simulink model "essai_5"  (R2016a)
settings: Solver=ode15s  StartTime=0.0  StopTime=1e9  RelTol=1e-3
libraries: nesl_utility x63, simCryogenics_lib x62, fl_lib x6
settings Model: Creator=FB229602  LastModifiedBy=FB229602
settings DataIOCC: LimitDataPoints=on  SaveFormat=Array
settings DebuggingCC: ParameterTunabilityLossMsg=none
settings HardwareCC: ProdBitPerInt=16  ProdBitPerPointer=16  ProdLargestAtomicFloat=None  ProdIntDivRoundTo=Undefined  ProdEndianess=Unspecified  ProdWordSize=16  ProdHWDeviceType=Generic->16-bit Embedded Processor  TargetBitPerPointer=64  TargetLongLongMode=on  TargetIntDivRoundTo=Zero  TargetEndianess=LittleEndian  TargetWordSize=64  TargetHWDeviceType=MATLAB Host  ProdEqTarget=off
settings ModelReferenceCC: PropagateSignalLabelsOutOfModel=off
settings ConfigComp: CovModelRefEnable=Off
settings SimscapeCC: SimscapeLogType=all

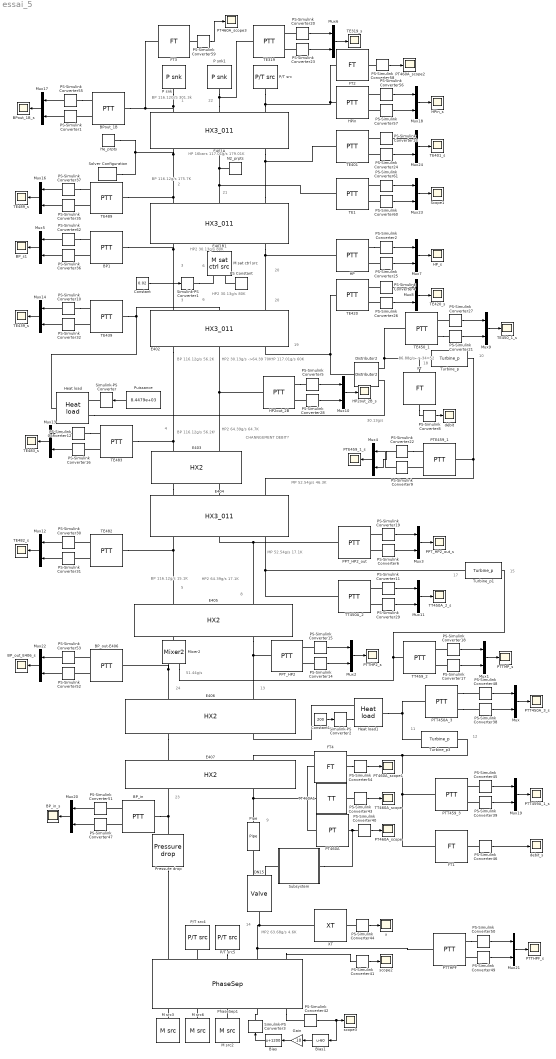
== system essai_5 ==
  note: 18
  note: 10
  note: 17
  note: 15
  note: 13
  note: 8
  note: 7
  note: 6
  note: 19
  note: 20
  note: 24
  note: 5
  note: 4
  note: 3
  note: MP
      | 52.54g/s
      | 17.1K
  note: HP2
      | 64.39g/s
      | 17.1K
  note: BP
      | 116.12g/s
      | 15.1K
  note: MP
      | 52.54g/s
      | 46.3K
  note: CHANNGEMENT DEBIT?
  note: HP2
      | 64.39g/s
      | 64.7K
  note: BP
      | 116.12g/s
      | 56.2K
  note: 30.13g/s
  note: 86.88g/s
      | ->-34=52
  note: HP
      | 117.01g/s
      | 60K
  note: HP2
      | 30.13g/s ->64.39
      | 70K
  note: BP
      | 116.12g/s
      | 56.2K
  note: HP2
      | 30.13g/s
      | 80K
  note: 51.44g/s
  note: 9
  note: 14
  note: 11
  note: 12
  note: 23
  note: MP2
      | 63.68g/s
      | 4.6K
  note: 6
  note: 20
  note: 21
  note: 22
  note: 3
  note: 2
  note: 1
  note: BP
      | 116.12G/S
      | 301.3k
  note: HP
      | 16bars
      | 117.01g/s
      | 179.01K
  note: BP
      | 116.12g/s
      | 175.7K
  note: HP2
      | 30.13g/s
      | 80K
  BP1 : simCryogenics_lib/Sensors/PTT
  BP_in : simCryogenics_lib/Sensors/PTT
  "BP_in_s " : Scope
  BP_out-E406 : simCryogenics_lib/Sensors/PTT
  BP_out_E406_s : Scope
  BP_s1 : Scope
  BPout_1B : simCryogenics_lib/Sensors/PTT
  BPout_1B_s : Scope
  Bias : Bias  Bias=1200
  Bias1 : Bias  Bias=-60
  Constant : Constant  Value=0.02
  Constant1 : Constant  Value=200
  "DN15 " : simCryogenics_lib/Elements/Valve  CVmax=1.5  ControlInputMin=0  ControlInputMax=100  Xt=0.86  Rv=10  lin_v=0  lim_v=0  K=2.4e-5 m^1.50000*kg^0.50000/s/bar^0.50000  Cmd_specify=off  Cmd_priority=High  Cmd=0  gamma_specify=off  gamma_priority=High  gamma=0  rho_specify=off  rho_priority=High  rho=0 kg/m^3  Xc_specify=off  Xc_priority=High  Xc=0  X_specify=off  X_priority=High  X=0  Y_specify=off  Y_priority=High  Y=0  CV_specify=off  CV_priority=High  CV=0
  Distributor2 : simCryogenics_lib/Elements/Distributor2
  E401A : simCryogenics_lib/Elements/HX3_011  N=9  Vh=0.118 m^3  Vm=0.055 m^3  Vc=0.008 km^3  M=281 kg  Kh=0.062/0.11612 s*bar/kg  Km=0.033/0.11701 s*bar/kg  Kc=0.021/0.11701 s*bar/kg  hh_m=0 J/s/K  hh_c=2.5e4 J/s/K  hm_c=250 J/s/K  Th0=300 K  Ph0=15 bar  Mh0=0.11612 kg/s  Tm0=175 K  Pm0=1 bar  Mm0=0.0026 kg/s  Tc0=175.7 K  Pc0=1.05 bar  Mc0=0.11612 kg/s  sensh=0  sensm=1  sensc=1
  E401B1 : simCryogenics_lib/Elements/HX3_011  N=9  Vh=0.133 m^3  Vm=0.062 m^3  Vc=0.012 m^3  M=195 kg  Kh=0.0255/0.11612 s*bar/kg  Km=0.014/0.11701 s*bar/kg  Kc=0.002/0.11701 s*bar/kg  hh_m=5000 J/s/K  hh_c=3e4 J/s/K  hm_c=1 J/s/K  Th0=179 K  Ph0=14.4 bar  Mh0=0.116 kg/s  Tm0=79 K  Pm0=1.1 bar  Mm0=0.0026 kg/s  Tc0=79.2 K  Pc0=1.05 bar  Mc0=0.116 kg/s  sensh=0  sensm=1  sensc=1
  E402 : simCryogenics_lib/Elements/HX3_011  N=9  Vh=0.133 m^3  Vm=0.005 m^3  Vc=0.012 m^3  M=195 kg  Kh=0.0255/0.11612 s*bar/kg  Km=0.011/0.03013 s*bar/kg  Kc=0.014/0.11701 s*bar/kg  hh_m=8000 J/s/K  hh_c=8000 J/s/K  hm_c=1 J/s/K  Th0=56.2 K  Ph0=1.05 bar  Mh0=0.11612 kg/s  Tm0=80 K  Pm0=14.73 bar  Mm0=0.06439 kg/s  Tc0=100 K  Pc0=14.73 bar  Mc0=0.11701 kg/s  sensh=0  sensm=1  sensc=1
  E403 : simCryogenics_lib/Elements/HX2  N=9  Vh=0.049 m^3  Vc=0.172 m^3  M=227.5 kg  Kh=0.003/0.06439 s*bar/kg  Kc=0.0055/0.11612 s*bar/kg  h=5700 J/s/K  Th0=64.7 K  Ph0=14.73 bar  Mh0=0.116 kg/s  Tc0=46 K  Pc0=1.05 bar  Mc0=0.064 kg/s
  E404 : simCryogenics_lib/Elements/HX3_011  N=9  Vh=0.172 m^3  Vm=0.049 m^3  Vc=0.045 m^3  M=227.5 kg  Kh=0.0055/0.011612 s*bar/kg  Km=0.003/0.06439 s*bar/kg  Kc=0.004/0.05254 s*bar/kg  hh_m=11000 J/s/K  hh_c=8000 J/s/K  hm_c=1 J/s/K  Th0=15.1 K  Ph0=1.05 bar  Mh0=0.116 kg/s  Tm0=46 K  Pm0=14.73 bar  Mm0=0.064 kg/s  Tc0=46.3 K  Pc0=5 bar  Mc0=0.052 kg/s  sensh=0  sensm=1  sensc=1
  "E405 " : simCryogenics_lib/Elements/HX2  N=9  Vh=0.023 m^3  Vc=0.065 m^3  M=64 kg  Kh=0.001/0.6439 s*bar/kg  Kc=0.0023/0.11612 s*bar/kg  h=1500 J/s/K  Th0=17.1 K  Ph0=14.73 bar  Mh0=0.11612 kg/s  Tc0=10 K  Pc0=1.05 bar  Mc0=0.06439 kg/s
  E406 : simCryogenics_lib/Elements/HX2  N=9  Vh=0.065 m^3  Vc=0.023 m^3  M=64 kg  Kh=0.001/0.06439 s*bar/kg  Kc=0.0023/0.06368 s*bar/kg  h=1000 J/s/K  Th0=17 K  Ph0=14.73 bar  Mh0=0.06368 kg/s  Tc0=5 K  Pc0=1.05 bar  Mc0=0.06439 kg/s
  E407 : simCryogenics_lib/Elements/HX2  N=9  Vh=0.011 m^3  Vc=0.065 m^3  M=64 kg  Kh=0.002/0.06368 s*bar/kg  Kc=0.0023/0.06368 s*bar/kg  h=2000 J/s/K  Th0=5.7 K  Ph0=3.03 bar  Mh0=0.06368 kg/s  Tc0=4.4 K  Pc0=1.05 bar  Mc0=0.06368 kg/s
  FT{,1..4} (5 alike) : simCryogenics_lib/Sensors/FT
  Gain : Gain  Gain=10
  HP : simCryogenics_lib/Sensors/PTT
  HP2out_2B : simCryogenics_lib/Sensors/PTT
  HP2out_2B_s : Scope
  HP_s : Scope
  HPin : simCryogenics_lib/Sensors/PTT
  HPin_s : Scope
  He_prpts : simCryogenics_lib/Utilities/He_prpts  P_min=0.1 bar  P_max=30 bar  T_min=3 K  T_max=320 K  N=100  Mol=4.0026 * 10 ^ (- 3) kg/mol
  Heat load : simCryogenics_lib/Utilities/Heat load
  Heat load1 : simCryogenics_lib/Utilities/Heat load
  M sat ctrl src : simCryogenics_lib/Sources_Sinks/M sat ctrl src
  M src2 : simCryogenics_lib/Sources_Sinks/M src  M=0 kg/s
  M src3 : simCryogenics_lib/Sources_Sinks/M src  M=0 kg/s
  M src6 : simCryogenics_lib/Sources_Sinks/M src  M=0 kg/s
  Mixer2 : simCryogenics_lib/Elements/Mixer2
  Mux{,1..14,16..24} (24 alike) : Mux  Inputs=2
  N2_prpts : simCryogenics_lib/Utilities/N2_prpts  P_min=0.5 bar  T_min=70 K  T_max=320 K  P_max=20 bar  Mol=4.0026 * (10 ^ (- 3)) kg/mol
  P snk : simCryogenics_lib/Sources_Sinks/P snk  P=1.05 bar
  P snk1 : simCryogenics_lib/Sources_Sinks/P snk  P=1.05 bar
  P/T src : simCryogenics_lib/Sources_Sinks/P//T src  P=14.73 bar  T=305 K
  P/T src4 : simCryogenics_lib/Sources_Sinks/P//T src  P=5 bar  T=46.3 K
  P/T src5 : simCryogenics_lib/Sources_Sinks/P//T src  P=5 bar  T=46.3 K
  PPT_HP2 : simCryogenics_lib/Sensors/PTT
  PPT_HP2_out : simCryogenics_lib/Sensors/PTT
  PPT_HP2_out_s : Scope
  PS Constant : fl_lib/Physical Signals/Sources/PS Constant  constant=0
  PS-Simulink Converter{1..2,4..6,8..32,35..62} (58 alike) : nesl_utility/PS-Simulink Converter  PhysicalDomain=network_engine_domain  SubClassName=ps_output  LeftPortType=input  RightPortType=output  PseudoPeriodic=off  Frequencies=[]  Unit=1  AffineConversion=off
  PT460A : simCryogenics_lib/Sensors/PT
  PT460A_scope{,1..3} (4 alike) : Scope
  PTE459_1 : simCryogenics_lib/Sensors/PTT
  PTE459_1_s : Scope
  PTT450A_3 : simCryogenics_lib/Sensors/PTT
  PTT450A_3_s : Scope
  PTT459A_1_s : Scope
  PTT459_3 : simCryogenics_lib/Sensors/PTT
  PTTHP2_s : Scope
  PTTHPF : simCryogenics_lib/Sensors/PTT
  PTTHPF_s : Scope
  PTTMP_s : Scope
  PhaseSep1 : simCryogenics_lib/Elements/PhaseSep  Ideal1=1  DeltaT1=0.05 K  N1=10  h1=400 W/K  Ideal2=1  DeltaT2=0.05 K  N2=10  h2=400 W/K  hmax=1.601 m  S=3.4636 m^2  P0=1.3 bar  h0=20  T0=4.5 K
  Pipe : simCryogenics_lib/Elements/Pipe  Vol=0.01 m^3  Ideal=0  P0=3 bar  T0=4.6 K
  Pressure drop : simCryogenics_lib/Utilities/Pressure drop  K=0.10/0.065 s*bar/kg
  "Puissance " : Constant  Value=8.4479e+03
  Scope1 : Scope
  Simulink-PS Converter{,1..3} (4 alike) : nesl_utility/Simulink-PS Converter  PhysicalDomain=network_engine_domain  SubClassName=ps_input  LeftPortType=input  RightPortType=output  PseudoPeriodic=off  Frequencies=[]  NoiseDistribution=none  NoiseParameters=[]  Unit=1  AffineConversion=off  InputFiltering=off  SimscapeFilterOrder=1  InputFilterTimeConstant=0.001  UdotUserProvided=1
  Solver Configuration : nesl_utility/Solver Configuration  PhysicalDomain=network_engine_domain  SubClassName=solver  LeftPortType=input  RightPortType=generic  Accelerate=off  Tones=[]  Harmonics=[]  SimulateNoise=off  Profile=off  UseLocalSampling=off  EnableSwitchedLinearOptims=on  FrequencyDomain=off  UseCCode=off  RelTol=0.001  AbsTol=1e-06  MinStep=1e-09  ToWorkspace=off  RevertToSquareIcSolve=off  NumHomotopyIterations=100  PhasorMode=off  PhasorModeNumHarmonics=1  OverrideAbsTol=off  DoDC=off  ResidualTolerance=1e-09  UseLocalSolver=off  LocalSolverChoice=NE_BACKWARD_EULER_ADVANCER  LocalSolverSampleTime=0.001  DoFixedCost=off  MaxNonlinIter=3  MaxModeIter=2  LinearAlgebra=Sparse  DelaysMemoryBudget=1024  AutomaticFiltering=on  FilteringTimeConstant=0.001
  Subsystem : Subsystem
  TE{1,319,401,420,439,482..483,489} (8 alike) : simCryogenics_lib/Sensors/PTT
  TE319_s : Scope
  TE401_s : Scope
  TE420_s : Scope
  TE439_s : Scope
  TE450_1 : simCryogenics_lib/Sensors/PTT
  TE450_1_s : Scope
  TE482_s : Scope
  TE483_s : Scope
  TE489_s : Scope
  TT450A_2 : simCryogenics_lib/Sensors/PTT
  TT450A_2_s : Scope
  TT459_2 : simCryogenics_lib/Sensors/PTT
  TT460A1 : simCryogenics_lib/Sensors/TT
  TT460A_scope : Scope
  Turbine_p : simCryogenics_lib/Elements/Turbine_p  A=2.5747e-05 m^2  D=0.05 m  Mass=0.02 kg  cst_eff=1  eta0=0.75  Tin0=60 K  Pin0=14.73 bar  Pout0=5 bar  N0=2250 1/s  Q0=0 W  v0=0  I=0 kg*m^2  gamma_specify=off  gamma_priority=High  gamma=0  C_specify=off  C_priority=High  C=0  Z_specify=off  Z_priority=High  Z=0  Cp_specify=off  Cp_priority=High  Cp=0 kJ/kg/K  Sin_specify=off  Sin_priority=High  Sin=0 kJ/kg  T_specify=off  T_priority=High  T=0 K  HoutIs_specify=off  HoutIs_priority=High  HoutIs=0 kJ/kg  u1_specify=off  u1_priority=High  u1=0 m/s  c1_specify=off  c1_priority=High  c1=0 m/s  v_specify=off  v_priority=High  v=0  eta_specify=off  eta_priority=High  eta=0  eta_var_specify=off  eta_var_priority=High  eta_var=0  N_specify=off  N_priority=High  N=0 rad/s  Q_specify=off  Q_priority=High  Q=0 W
  Turbine_p1 : simCryogenics_lib/Elements/Turbine_p  A=2.6523e-05 m^2  D=0.02 m  Mass=0.02 kg  cst_eff=1  eta0=0.75  Tin0=17.1 K  Pin0=5 bar  Pout0=1.3 bar  N0=2250 1/s  Q0=0 W  v0=0  I=0 kg*m^2  gamma_specify=off  gamma_priority=High  gamma=0  C_specify=off  C_priority=High  C=0  Z_specify=off  Z_priority=High  Z=0  Cp_specify=off  Cp_priority=High  Cp=0 kJ/kg/K  Sin_specify=off  Sin_priority=High  Sin=0 kJ/kg  T_specify=off  T_priority=High  T=0 K  HoutIs_specify=off  HoutIs_priority=High  HoutIs=0 kJ/kg  u1_specify=off  u1_priority=High  u1=0 m/s  c1_specify=off  c1_priority=High  c1=0 m/s  v_specify=off  v_priority=High  v=0  eta_specify=off  eta_priority=High  eta=0  eta_var_specify=off  eta_var_priority=High  eta_var=0  N_specify=off  N_priority=High  N=0 rad/s  Q_specify=off  Q_priority=High  Q=0 W
  Turbine_p3 : simCryogenics_lib/Elements/Turbine_p  A=6.0851e-06 m^2  D=0.01 m  Mass=0.02 kg  cst_eff=0  eta0=0.75  Tin0=7.19 K  Pin0=14.73 bar  Pout0=3.03 bar  N0=2250 1/s  Q0=0 W  v0=0  I=0 kg*m^2  gamma_specify=off  gamma_priority=High  gamma=0  C_specify=off  C_priority=High  C=0  Z_specify=off  Z_priority=High  Z=0  Cp_specify=off  Cp_priority=High  Cp=0 kJ/kg/K  Sin_specify=off  Sin_priority=High  Sin=0 kJ/kg  T_specify=off  T_priority=High  T=0 K  HoutIs_specify=off  HoutIs_priority=High  HoutIs=0 kJ/kg  u1_specify=off  u1_priority=High  u1=0 m/s  c1_specify=off  c1_priority=High  c1=0 m/s  v_specify=off  v_priority=High  v=0  eta_specify=off  eta_priority=High  eta=0  eta_var_specify=off  eta_var_priority=High  eta_var=0  N_specify=off  N_priority=High  N=0 rad/s  Q_specify=off  Q_priority=High  Q=0 W
  XT : simCryogenics_lib/Sensors/XT
  debit_s : Scope
  débit : Scope
  scope2 : Scope
  scope3 : Scope
  x : Scope
  wires:
  "Puissance "/1 -> Simulink-PS Converter/1
  PS-Simulink Converter8/1 -> débit/1
  PS-Simulink Converter15/1 -> Mux2/1
  PS-Simulink Converter14/1 -> Mux2/2
  Mux2/1 -> PTTHP2_s/1
  PS-Simulink Converter18/1 -> Mux1/1
  PS-Simulink Converter17/1 -> Mux1/2
  Mux1/1 -> PTTMP_s/1
  PS-Simulink Converter19/1 -> Mux3/1
  PS-Simulink Converter6/1 -> Mux3/2
  Mux3/1 -> PPT_HP2_out_s/1
  Mux4/1 -> PTE459_1_s/1
  PS-Simulink Converter25/1 -> Mux7/2
  Mux7/1 -> HP_s/1
  PS-Simulink Converter4/1 -> Mux8/1
  PS-Simulink Converter26/1 -> Mux8/2
  Mux8/1 -> TE420_s/1
  PS-Simulink Converter27/1 -> Mux9/1
  Mux9/1 -> TE450_1_s/1
  PS-Simulink Converter2/1 -> Mux7/1
  PS-Simulink Converter28/1 -> Mux10/2
  Mux10/1 -> HP2out_2B_s/1
  PS-Simulink Converter5/1 -> Mux10/1
  PS-Simulink Converter11/1 -> Mux11/1
  PS-Simulink Converter29/1 -> Mux11/2
  Mux11/1 -> TT450A_2_s/1
  Mux12/1 -> TE482_s/1
  PS-Simulink Converter30/1 -> Mux12/1
  PS-Simulink Converter31/1 -> Mux12/2
  Mux13/1 -> TE483_s/1
  PS-Simulink Converter12/1 -> Mux13/1
  PS-Simulink Converter16/1 -> Mux13/2
  Mux14/1 -> TE439_s/1
  PS-Simulink Converter10/1 -> Mux14/1
  PS-Simulink Converter32/1 -> Mux14/2
  PS-Simulink Converter9/1 -> Mux4/1
  PS-Simulink Converter22/1 -> Mux4/2
  PS-Simulink Converter21/1 -> Mux9/2
  Bias/1 -> Simulink-PS Converter3/1
  PS-Simulink Converter46/1 -> debit_s/1
  PS-Simulink Converter40/1 -> PT460A_scope/1
  PS-Simulink Converter43/1 -> TT460A_scope/1
  PS-Simulink Converter44/1 -> x/1
  PS-Simulink Converter48/1 -> Mux/1
  PS-Simulink Converter42/1 -> Bias1/1, scope3/1
  Gain/1 -> Bias/1
  Bias1/1 -> Gain/1
  PS-Simulink Converter38/1 -> Mux/2
  Mux/1 -> PTT450A_3_s/1
  PS-Simulink Converter45/1 -> Mux19/1
  PS-Simulink Converter39/1 -> Mux19/2
  Mux19/1 -> PTT459A_1_s/1
  PS-Simulink Converter50/1 -> Mux21/1
  PS-Simulink Converter49/1 -> Mux21/2
  Mux21/1 -> PTTHPF_s/1
  Mux20/1 -> "BP_in_s "/1
  PS-Simulink Converter51/1 -> Mux20/1
  PS-Simulink Converter47/1 -> Mux20/2
  Mux22/1 -> BP_out_E406_s/1
  PS-Simulink Converter53/1 -> Mux22/1
  PS-Simulink Converter52/1 -> Mux22/2
  PS-Simulink Converter41/1 -> scope2/1
  PS-Simulink Converter54/1 -> PT460A_scope1/1
  PS-Simulink Converter20/1 -> Mux6/1
  PS-Simulink Converter23/1 -> Mux6/2
  Mux6/1 -> TE319_s/1
  PS-Simulink Converter13/1 -> Mux24/1
  PS-Simulink Converter24/1 -> Mux24/2
  Mux24/1 -> TE401_s/1
  Mux5/1 -> BP_s1/1
  PS-Simulink Converter62/1 -> Mux5/1
  PS-Simulink Converter36/1 -> Mux5/2
  Mux16/1 -> TE489_s/1
  PS-Simulink Converter37/1 -> Mux16/1
  PS-Simulink Converter35/1 -> Mux16/2
  Mux17/1 -> BPout_1B_s/1
  PS-Simulink Converter55/1 -> Mux17/1
  PS-Simulink Converter1/1 -> Mux17/2
  PS-Simulink Converter56/1 -> Mux18/1
  PS-Simulink Converter57/1 -> Mux18/2
  Mux18/1 -> HPin_s/1
  PS-Simulink Converter58/1 -> PT460A_scope2/1
  PS-Simulink Converter59/1 -> PT460A_scope3/1
  PS-Simulink Converter60/1 -> Mux23/2
  Mux23/1 -> Scope1/1
  PS-Simulink Converter61/1 -> Mux23/1
  Constant/1 -> Simulink-PS Converter1/1
  Constant1/1 -> Simulink-PS Converter2/1
  connections:
  "E405 "/LConn1 -- E404/LConn3 -- TE482/LConn1
  E402/LConn3 -- E403/LConn1 -- TE483/LConn1
  E402/LConn2 -- E403/LConn2 -- HP2out_2B/LConn1
  "E405 "/LConn2 -- E404/LConn2 -- PPT_HP2_out/LConn1
  TT450A_2/LConn1 -- E404/LConn1 -- Turbine_p1/LConn1
  Turbine_p/RConn1 -- E404/RConn1 -- PTE459_1/LConn1
  E401B1/RConn1 -- E402/RConn3 -- BP1/LConn1
  HP/LConn1 -- E401B1/RConn3 -- E402/RConn1
  Distributor2/LConn1 -- TE420/LConn1 -- E402/LConn1
  Heat load/RConn1 -- TE439/LConn1 -- E402/RConn2
  FT/LConn1 -- TE450_1/LConn1 -- Distributor2/RConn1 -- Turbine_p/LConn1
  Heat load/LConn1 -- Distributor2/RConn2
  Simulink-PS Converter/RConn1 -- Heat load/LConn2
  FT/RConn1 -- PS-Simulink Converter8/LConn1
  Mixer2/RConn1 -- "E405 "/RConn1
  Mixer2/LConn2 -- TT459_2/LConn1 -- Turbine_p1/RConn1
  PS-Simulink Converter14/LConn1 -- PPT_HP2/RConn2
  PS-Simulink Converter15/LConn1 -- PPT_HP2/RConn1
  PS-Simulink Converter17/LConn1 -- TT459_2/RConn2
  PS-Simulink Converter18/LConn1 -- TT459_2/RConn1
  PS-Simulink Converter19/LConn1 -- PPT_HP2_out/RConn1
  PS-Simulink Converter6/LConn1 -- PPT_HP2_out/RConn2
  PS-Simulink Converter22/LConn1 -- PTE459_1/RConn2
  PTE459_1/RConn1 -- PS-Simulink Converter9/LConn1
  PS-Simulink Converter25/LConn1 -- HP/RConn2
  PS-Simulink Converter4/LConn1 -- TE420/RConn1
  PS-Simulink Converter26/LConn1 -- TE420/RConn2
  PS-Simulink Converter27/LConn1 -- TE450_1/RConn1
  HP/RConn1 -- PS-Simulink Converter2/LConn1
  HP2out_2B/RConn1 -- PS-Simulink Converter5/LConn1
  PS-Simulink Converter28/LConn1 -- HP2out_2B/RConn2
  PS-Simulink Converter29/LConn1 -- TT450A_2/RConn2
  PS-Simulink Converter11/LConn1 -- TT450A_2/RConn1
  TE450_1/RConn2 -- PS-Simulink Converter21/LConn1
  TE482/RConn1 -- PS-Simulink Converter30/LConn1
  TE482/RConn2 -- PS-Simulink Converter31/LConn1
  TE483/RConn2 -- PS-Simulink Converter16/LConn1
  PS-Simulink Converter12/LConn1 -- TE483/RConn1
  TE439/RConn2 -- PS-Simulink Converter32/LConn1
  PS-Simulink Converter10/LConn1 -- TE439/RConn1
  E407/RConn1 -- Pressure drop/RConn1 -- BP_in/LConn1
  PT460A/LConn1 -- FT4/LConn1 -- E407/RConn2 -- Pipe/LConn1 -- TT460A1/LConn1
  PTT450A_3/LConn1 -- Turbine_p3/LConn1 -- Heat load1/RConn1
  PTT459_3/LConn1 -- FT1/LConn1 -- Turbine_p3/RConn1 -- E407/LConn2
  "DN15 "/RConn1 -- PhaseSep1/LConn4 -- PTTHPF/LConn1 -- XT/LConn1
  PhaseSep1/LConn5 -- PS-Simulink Converter41/LConn1
  BP_in/RConn1 -- PS-Simulink Converter51/LConn1
  BP_out-E406/RConn1 -- PS-Simulink Converter53/LConn1
  PS-Simulink Converter44/LConn1 -- XT/RConn1
  PT460A/RConn1 -- Subsystem/RConn1 -- PS-Simulink Converter40/LConn1
  E406/RConn1 -- E407/LConn1
  PhaseSep1/LConn2 -- P/T src4/RConn1
  M src2/RConn1 -- PhaseSep1/RConn3
  BP_in/RConn2 -- PS-Simulink Converter47/LConn1
  "E405 "/RConn2 -- E406/LConn2 -- PPT_HP2/LConn1
  P/T src5/RConn1 -- PhaseSep1/LConn3
  PS-Simulink Converter39/LConn1 -- PTT459_3/RConn2
  PS-Simulink Converter46/LConn1 -- FT1/RConn1
  PS-Simulink Converter49/LConn1 -- PTTHPF/RConn2
  PTT450A_3/RConn1 -- PS-Simulink Converter48/LConn1
  PS-Simulink Converter43/LConn1 -- TT460A1/RConn1
  "DN15 "/LConn2 -- Pipe/RConn1
  M src6/RConn1 -- PhaseSep1/RConn2
  Simulink-PS Converter3/RConn1 -- PhaseSep1/RConn4
  PhaseSep1/RConn5 -- PS-Simulink Converter42/LConn1
  M src3/RConn1 -- PhaseSep1/RConn1
  PS-Simulink Converter45/LConn1 -- PTT459_3/RConn1
  PTT450A_3/RConn2 -- PS-Simulink Converter38/LConn1
  E406/LConn1 -- BP_out-E406/LConn1 -- Mixer2/LConn1
  E403/RConn1 -- E404/RConn3
  E403/RConn2 -- E404/RConn2
  BP_out-E406/RConn2 -- PS-Simulink Converter52/LConn1
  PTTHPF/RConn1 -- PS-Simulink Converter50/LConn1
  Pressure drop/LConn1 -- PhaseSep1/LConn1
  FT4/RConn1 -- PS-Simulink Converter54/LConn1
  Subsystem/LConn1 -- "DN15 "/LConn1
  FT3/LConn1 -- BPout_1B/LConn1 -- P snk/RConn1 -- E401A/LConn1
  E401A/RConn1 -- He_prpts/RConn1 -- Solver Configuration/RConn1 -- E401B1/LConn1 -- TE489/LConn1
  E401A/LConn3 -- FT2/LConn1 -- HPin/LConn1 -- P/T src/RConn1
  E401B1/LConn3 -- E401A/RConn3 -- TE401/LConn1
  E401A/LConn2 -- TE319/LConn1 -- P snk1/RConn1
  N2_prpts/RConn1 -- E401A/RConn2 -- E401B1/LConn2 -- TE1/LConn1
  PS-Simulink Converter56/LConn1 -- HPin/RConn1
  PS-Simulink Converter13/LConn1 -- TE401/RConn1
  BPout_1B/RConn2 -- PS-Simulink Converter1/LConn1
  PS-Simulink Converter37/LConn1 -- TE489/RConn1
  PS-Simulink Converter23/LConn1 -- TE319/RConn2
  PS-Simulink Converter60/LConn1 -- TE1/RConn2
  PS-Simulink Converter61/LConn1 -- TE1/RConn1
  PS-Simulink Converter20/LConn1 -- TE319/RConn1
  PS-Simulink Converter59/LConn1 -- FT3/RConn1
  PS-Simulink Converter24/LConn1 -- TE401/RConn2
  PS-Simulink Converter55/LConn1 -- BPout_1B/RConn1
  TE489/RConn2 -- PS-Simulink Converter35/LConn1
  M sat ctrl src/RConn1 -- E401B1/RConn2
  PS-Simulink Converter57/LConn1 -- HPin/RConn2
  PS-Simulink Converter58/LConn1 -- FT2/RConn1
  PS-Simulink Converter62/LConn1 -- BP1/RConn1
  BP1/RConn2 -- PS-Simulink Converter36/LConn1
  Simulink-PS Converter1/RConn1 -- M sat ctrl src/LConn1
  PS Constant/RConn1 -- M sat ctrl src/LConn2
  Heat load1/LConn1 -- E406/RConn2
  Simulink-PS Converter2/RConn1 -- Heat load1/LConn2

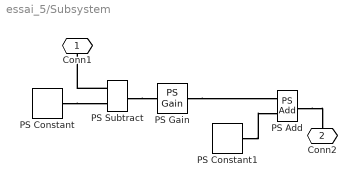
== system essai_5/Subsystem ==
  PS Add : fl_lib/Physical Signals/Functions/PS Add
  PS Constant : fl_lib/Physical Signals/Sources/PS Constant  constant=3
  PS Constant1 : fl_lib/Physical Signals/Sources/PS Constant  constant=63
  PS Gain : fl_lib/Physical Signals/Functions/PS Gain  gain=85
  PS Subtract : fl_lib/Physical Signals/Functions/PS Subtract
  Conn1 : PMIOPort  Port=1  Side=Right
  Conn2 : PMIOPort  Port=2  Side=Left
  connections:
  PS Constant/RConn1 -- PS Subtract/LConn2
  PS Subtract/RConn1 -- PS Gain/LConn1
  PS Gain/RConn1 -- PS Add/LConn1
  PS Subtract/LConn1 -- Conn1/RConn1
  PS Constant1/RConn1 -- PS Add/LConn2
  PS Add/RConn1 -- Conn2/RConn1
